simulink model "ServoMotor"  (R2024a)
settings: Solver=ode15s  StartTime=0.0  StopTime=10.0  RelTol=1e-3
model workspace (MAT data in the model file):
  J = 5e-05
  L = 0.01
  R = 4
  b = 0.0005
  k = 0.2
  ki = 7.33
  kp = 9.39
  ts = 0.1
  v = 7.4
settings Model: Creator=awabm  LastModifiedBy=awabm

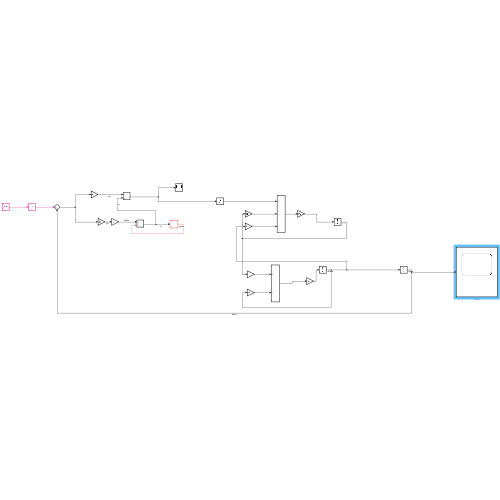
[thumbnail: Simulink's stored preview of the top-level diagram]
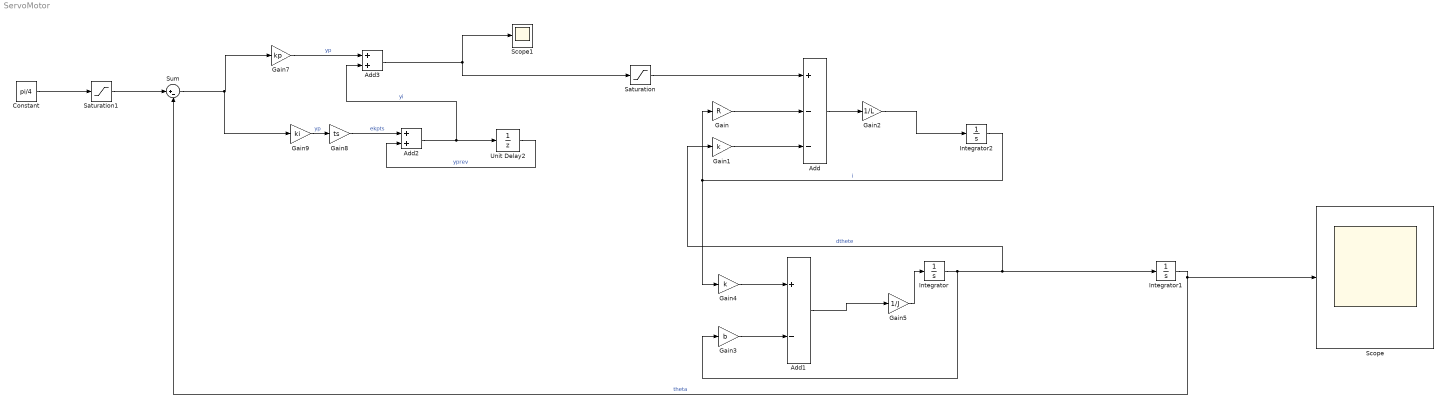
== system ServoMotor ==
  Add : Sum  Inputs=+--
  Add1 : Sum  Inputs=+-
  Add2 : Sum
  Add3 : Sum
  Constant : Constant  Value=pi/4
  Gain : Gain  Gain=R
  Gain1 : Gain  Gain=k
  Gain2 : Gain  Gain=1/L
  Gain3 : Gain  Gain=b
  Gain4 : Gain  Gain=k
  Gain5 : Gain  Gain=1/J
  Gain7 : Gain  Gain=kp
  Gain8 : Gain  Gain=ts
  Gain9 : Gain  Gain=ki
  Integrator : Integrator
  Integrator1 : Integrator
  Integrator2 : Integrator
  Saturation : Saturate  UpperLimit=v  LowerLimit=-v
  Saturation1 : Saturate  UpperLimit=pi/4  LowerLimit=-pi/4
  Scope : Scope
  Scope1 : Scope
  Sum : Sum  Inputs=|+-
  Unit Delay2 : UnitDelay  SampleTime=ts  HasFrameUpgradeWarning=on
  wires:
  Add3/1 -> Saturation/1, Scope1/1
  Gain/1 -> Add/2
  Gain1/1 -> Add/3
  Add/1 -> Gain2/1
  Integrator/1 -> Gain3/1, Integrator1/1, Gain1/1  "dthete"
  Gain3/1 -> Add1/2
  Gain4/1 -> Add1/1
  Integrator2/1 -> Gain4/1, Gain/1  "i"
  Add1/1 -> Gain5/1
  Gain2/1 -> Integrator2/1
  Gain5/1 -> Integrator/1
  Integrator1/1 -> Sum/2, Scope/1  "theta"
  Gain7/1 -> Add3/1  "yp"
  Gain8/1 -> Add2/1  "ekpts"
  Unit Delay2/1 -> Add2/2  "yprev"
  Gain9/1 -> Gain8/1  "yp"
  Add2/1 -> Add3/2, Unit Delay2/1  "yi"
  Constant/1 -> Saturation1/1
  Sum/1 -> Gain9/1, Gain7/1
  Saturation/1 -> Add/1
  Saturation1/1 -> Sum/1
